simulink model "modulation"  (R2013a)
settings: Solver=ode45  StartTime=0.0  StopTime=10.0  RelTol=1e-3
values from neighbouring files (symbols this model uses):
  i = i+2    (= 3)    [QPSK_sim1.m]
  lengthOfSymbol = 64    [GSM_sim_ISI_config.m]    (also in GSM_sim_config.m; modulationsarten_config.m)
  sampleTime = 1    [GSM_sim_ISI_config.m]    (also in GSM_sim_config.m; modulationsarten_config.m)
libraries: commchan3 x5, commdigbbndcpm2 x3, commutil2 x2, commdigbbndam3 x1, commdigbbndpm3 x1, dspsigops x1
settings Model: Creator=mainster  LastModifiedBy=mainster
settings DataIOCC: SignalLoggingSaveFormat=ModelDataLogs
settings OptimizationCC: ExpressionDepthLimit=2147483647
settings DebuggingCC: SolverPrmCheckMsg=none  FcnCallInpInsideContextMsg=UseLocalSettings
settings GRTTargetCC: CombineOutputUpdateFcns=off  GRTInterface=on

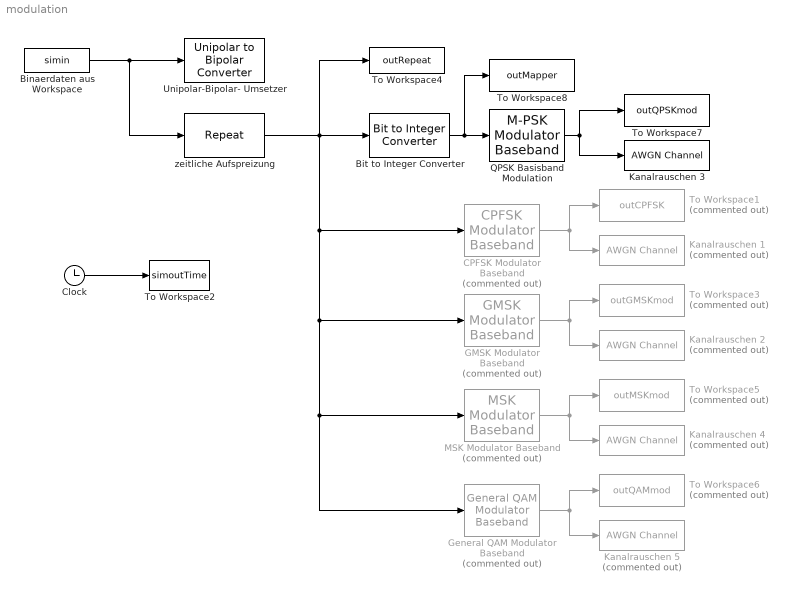
== system modulation ==
  Binaerdaten aus Workspace : FromWorkspace  VariableName=simin  SampleTime=sampleTime
  Bit to Integer Converter : commutil2/Bit to Integer Converter  nbits=2  bitOrder=MSB first  signedOutputValues=Unsigned  outDtype=Inherit via internal rule  outDtypeSigned=Inherit via internal rule
  CPFSK Modulator Baseband : commdigbbndcpm2/CPFSK Modulator Baseband  Commented=on  Mnum=4  inputType=Integer  mappingType=Binary  modIdx=.5  phaseOffset=0  samplesPerSymbol=8  RateOptions=Enforce single-rate processing  outDataType=double
  Clock : Clock
  GMSK Modulator Baseband : commdigbbndcpm2/GMSK Modulator Baseband  Commented=on  inputType=Integer  BT=.3  pulseLength=4  preHistory=1  phaseOffset=0  samplesPerSymbol=8  RateOptions=Enforce single-rate processing  outDataType=double
  General QAM Modulator Baseband : commdigbbndam3/General QAM Modulator Baseband  Commented=on  SigCon=[exp(2*pi*i*[0:7]/8)]  outDtype=double  outWordLen=16  outUDDataType=sfix(16)  outFracLenMode=Best precision  outFracLen=15
  Kanalrauschen {1..2,4..5} (4 alike) : commchan3/AWGN Channel  Commented=on  InputProcessing=Inherited (this choice will be removed - see release notes)  seed=67  noiseMode="Signal to noise ratio  (SNR)"  EbNodB=30  EsNodB=10  SNRdB=SNR  bitsPerSym=1  Ps=1  Tsym=1  variance=1
  Kanalrauschen 3 : commchan3/AWGN Channel  InputProcessing=Inherited (this choice will be removed - see release notes)  seed=67  noiseMode="Signal to noise ratio  (SNR)"  EbNodB=30  EsNodB=10  SNRdB=SNR  bitsPerSym=1  Ps=1  Tsym=1  variance=1
  MSK Modulator Baseband : commdigbbndcpm2/MSK Modulator Baseband  Commented=on  inputType=Integer  phaseOffset=0  samplesPerSymbol=8  RateOptions=Enforce single-rate processing  outDataType=double
  QPSK Basisband Modulation : commdigbbndpm3/M-PSK Modulator Baseband  M=4  InType=Integer  Enc=Gray  Mapping=[0:2]  Ph=phaseOffset  outDtype=double  outWordLen=16  outUDDataType=sfix(16)  outFracLenMode=Best precision  outFracLen=15
  To Workspace1 : ToWorkspace  Commented=on  VariableName=outCPFSK  SampleTime=-1  SaveFormat=Structure
  To Workspace2 : ToWorkspace  VariableName=simoutTime  SampleTime=-1  SaveFormat=Structure
  To Workspace3 : ToWorkspace  Commented=on  VariableName=outGMSKmod  SampleTime=-1  SaveFormat=Structure
  To Workspace4 : ToWorkspace  VariableName=outRepeat  SampleTime=-1  SaveFormat=Structure
  To Workspace5 : ToWorkspace  Commented=on  VariableName=outMSKmod  SampleTime=-1  SaveFormat=Structure
  To Workspace6 : ToWorkspace  Commented=on  VariableName=outQAMmod  SampleTime=-1  SaveFormat=Structure
  To Workspace7 : ToWorkspace  VariableName=outQPSKmod  SampleTime=-1  SaveFormat=Structure
  To Workspace8 : ToWorkspace  VariableName=outMapper  SampleTime=-1  SaveFormat=Structure
  Unipolar-Bipolar- Umsetzer : commutil2/Unipolar to Bipolar Converter  M=2  polarity=Positive  dataType=Inherit via internal rule
  zeitliche Aufspreizung : dspsigops/Repeat  N=lengthOfSymbol  InputProcessing=Inherited (this choice will be removed - see release notes)  RateOptions=Allow multirate processing  ic=0  mode=Unused parameter value
  wires:
  Binaerdaten aus Workspace/1 -> Unipolar-Bipolar- Umsetzer/1, zeitliche Aufspreizung/1
  Clock/1 -> To Workspace2/1
  QPSK Basisband Modulation/1 -> Kanalrauschen 3/1, To Workspace7/1
  zeitliche Aufspreizung/1 -> Bit to Integer Converter/1, General QAM Modulator Baseband/1, MSK Modulator Baseband/1, GMSK Modulator Baseband/1, CPFSK Modulator Baseband/1, To Workspace4/1
  CPFSK Modulator Baseband/1 -> Kanalrauschen 1/1, To Workspace1/1
  GMSK Modulator Baseband/1 -> To Workspace3/1, Kanalrauschen 2/1
  MSK Modulator Baseband/1 -> Kanalrauschen 4/1, To Workspace5/1
  General QAM Modulator Baseband/1 -> Kanalrauschen 5/1, To Workspace6/1
  Bit to Integer Converter/1 -> To Workspace8/1, QPSK Basisband Modulation/1
